simulink model "spm_running"  (R2016a)
settings: Solver=VariableStepAuto  StartTime=0.0  StopTime=2  MaxStep=1e-3
values from neighbouring files (symbols this model uses):
  alpha_0 = deg2rad(68)    [spm_running_setup.m]
  g = 9.81    [spm_running_setup.m]
  k = 20000    [spm_running_setup.m]
  l_0 = 1    [spm_running_setup.m]
  m = 80    [spm_running_setup.m]
  xdot_0 = 5    [spm_running_setup.m]
  y_0 = 1    [spm_running_setup.m]
settings Model: Creator=Cyrus  LastModifiedBy=Cyrus
settings GRTTargetCC: GeneratePreprocessorConditionals=Use local settings

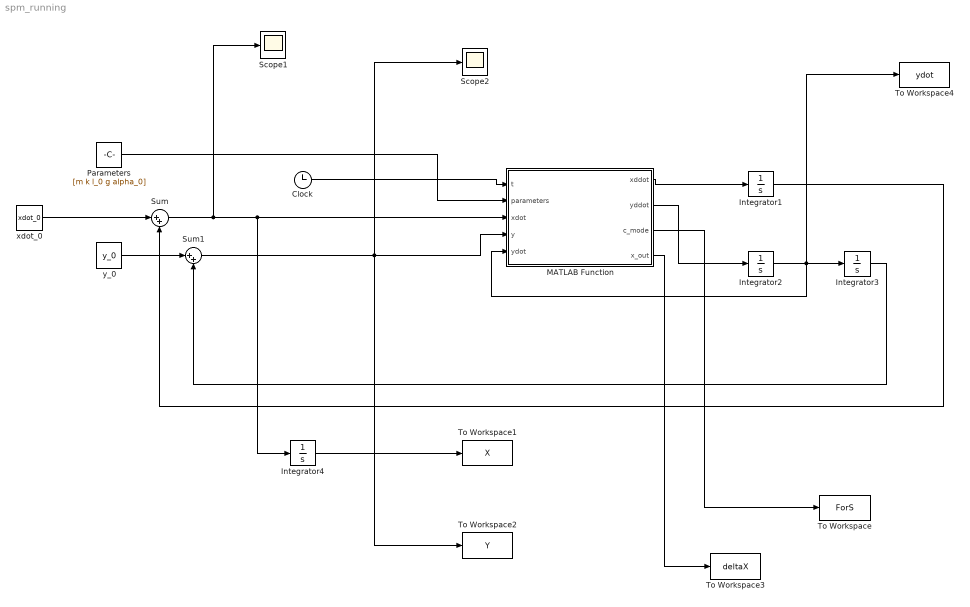
== system spm_running ==
  Clock : Clock
  Integrator{1..4} (4 alike) : Integrator
  MATLAB Function : MATLAB Function  TreatAsAtomicUnit=on
  Parameters : Constant  Value=[m k l_0 g alpha_0]
  Scope1 : Scope
  Scope2 : Scope
  Sum : Sum  Inputs=|++
  Sum1 : Sum  Inputs=|++
  To Workspace : ToWorkspace  VariableName=ForS  SaveFormat=Timeseries  SampleTime=-1
  To Workspace1 : ToWorkspace  VariableName=X  SaveFormat=Timeseries  SampleTime=-1
  To Workspace2 : ToWorkspace  VariableName=Y  SaveFormat=Timeseries  SampleTime=-1
  To Workspace3 : ToWorkspace  VariableName=deltaX  SaveFormat=Timeseries  SampleTime=-1
  To Workspace4 : ToWorkspace  VariableName=ydot  SaveFormat=Timeseries  SampleTime=-1
  xdot_0 : Constant  Value=xdot_0
  y_0 : Constant  Value=y_0
  wires:
  Parameters/1 -> MATLAB Function/2(parameters)
  MATLAB Function/1(xddot) -> Integrator1/1
  Integrator1/1 -> Sum/2
  xdot_0/1 -> Sum/1
  Sum/1 -> Scope1/1, MATLAB Function/3(xdot), Integrator4/1
  MATLAB Function/2(yddot) -> Integrator2/1
  y_0/1 -> Sum1/1
  Integrator3/1 -> Sum1/2
  Sum1/1 -> To Workspace2/1, Scope2/1, MATLAB Function/4(y)
  Clock/1 -> MATLAB Function/1(t)
  Integrator2/1 -> To Workspace4/1, MATLAB Function/5(ydot), Integrator3/1
  MATLAB Function/3(c_mode) -> To Workspace/1
  Integrator4/1 -> To Workspace1/1
  MATLAB Function/4(x_out) -> To Workspace3/1

== matlab function spm_running/MATLAB Function ==
  data: t input; parameters input; xdot input; xddot output; yddot output; y input; c_mode output; ydot input; x_out output
function [xddot, yddot, c_mode, x_out] = fcn(t, parameters, xdot, y, ydot)
%#codegen
m = parameters(1);
k = parameters(2);
l_0 = parameters(3);
g = parameters(4);
alpha_0 = parameters(5);



persistent mode;
persistent x;
persistent time;

if isempty(mode) 
    mode = 0;
end

if isempty(x) 
    x = -l_0*cos(alpha_0);
end

if isempty(time) 
    time = 0;
end

l = sqrt(x.^2+y.^2);
if mode == 1
    if l >= l_0
        mode = 0;
        x = -l_0*cos(alpha_0);
    end
else
    if y <= l_0*sin(alpha_0) && ydot<=0;
        mode = 1;
        time = t;
    end
end


if mode == 1
    x = x+xdot*(t-time);
    l = sqrt(x.^2+y.^2);
    xddot = (k*(l_0/l -1)*x)/m;
    yddot = (k*(l_0/l -1)*y)/m-g;
    time = t;
else
    xddot = 0;
    yddot = -g;
end

c_mode = mode;
x_out = x;
